simulink model "four"  (R2014a)
settings: Solver=ode45  StartTime=0.0  StopTime=30  MaxStep=0.001  MinStep=0.0001  RelTol=1e-3
libraries: simulink x2
settings Model: Creator=Valentin  LastModifiedBy=trigg

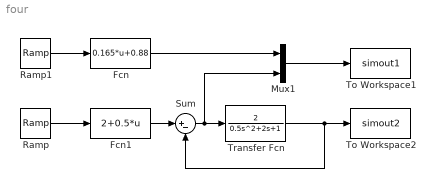
== system four ==
  Fcn : Fcn  Expr=0.165*u+0.88
  Fcn1 : Fcn  Expr=2+0.5*u
  Mux1 : Mux  Inputs=2
  Ramp : simulink/Sources/Ramp  slope=1  start=0  X0=0
  Ramp1 : simulink/Sources/Ramp  slope=1  start=0  X0=0
  Sum : Sum  Inputs=|+-
  To Workspace1 : ToWorkspace  VariableName=simout1  SaveFormat=Timeseries  SampleTime=-1
  To Workspace2 : ToWorkspace  VariableName=simout2  SaveFormat=Timeseries  SampleTime=-1
  Transfer Fcn : TransferFcn  Numerator=[2]  Denominator=[0.5 2 1]
  wires:
  Sum/1 -> Transfer Fcn/1, Mux1/2
  Transfer Fcn/1 -> To Workspace2/1, Sum/2
  Fcn1/1 -> Sum/1
  Fcn/1 -> Mux1/1
  Ramp1/1 -> Fcn/1
  Ramp/1 -> Fcn1/1
  Mux1/1 -> To Workspace1/1
